simulink model "pidmodel"  (R2013b)
settings: Solver=ode45  StartTime=0.0  StopTime=10  RelTol=1e-3
InitFcn:
  | param
undefined symbols (not defined in the file or in its folder): AP, can_ctrl
settings Model: Creator=paul  LastModifiedBy=paul

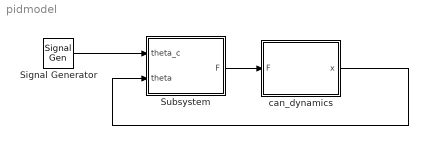
== system pidmodel ==
  Signal Generator : SignalGenerator  WaveForm=square  Amplitude=pi/3
  Subsystem : Subsystem
  can_dynamics : Subsystem
  wires:
  Signal Generator/1 -> Subsystem/1(theta_c)
  can_dynamics/1(x) -> Subsystem/2(theta)
  Subsystem/1(F) -> can_dynamics/1(F)

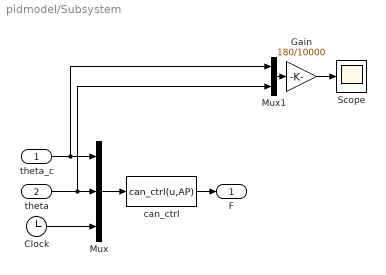
== system pidmodel/Subsystem ==
  theta_c : Inport
  theta : Inport  Port=2
  Clock : Clock
  Gain : Gain  Gain=180/10000
  Mux : Mux  Inputs=3
  Mux1 : Mux  Inputs=2
  Scope : Scope
      settings: TimeRange=10  YMin=-0.025  YMax=0.025
  can_ctrl : MATLABFcn  MATLABFcn=can_ctrl(u,AP)  OutputDimensions=1  SampleTime=AP.Ts
  F : Outport
  wires:
  theta_c/1 -> Mux1/1, Mux/1
  Mux/1 -> can_ctrl/1
  Gain/1 -> Scope/1
  Mux1/1 -> Gain/1
  can_ctrl/1 -> F/1
  Clock/1 -> Mux/3
  theta/1 -> Mux1/2, Mux/2

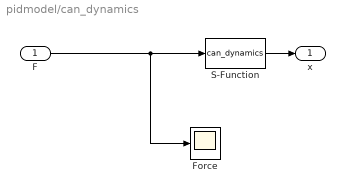
== system pidmodel/can_dynamics ==
  F : Inport
  Force : Scope
      settings: TimeRange=10  YMin=-0.08  YMax=0.08
  S-Function : S-Function  FunctionName=can_dynamics  Parameters=AP  EnableBusSupport=off
  x : Outport
  wires:
  F/1 -> Force/1, S-Function/1
  S-Function/1 -> x/1
